simulink model "Fuzzy"  (R2021a)
settings: Solver=VariableStepAuto  StartTime=0.0  StopTime=30  RelTol=1e-3
values from neighbouring files (symbols this model uses):
  K = Kp/(a*Ke)    (= 32)    [code.m]    (also in tester.m)
  Kd = a*Ke    (= 0.0566666666667)    [code.m]    (also in tester.m = 0.0416666666667)
  Ke = 1.5    [code.m]    (also in tester.m)
libraries: simulink x3, fuzblock x1
settings Model: PauseTimes=10  Creator=Administrator  LastModifiedBy=Administrator

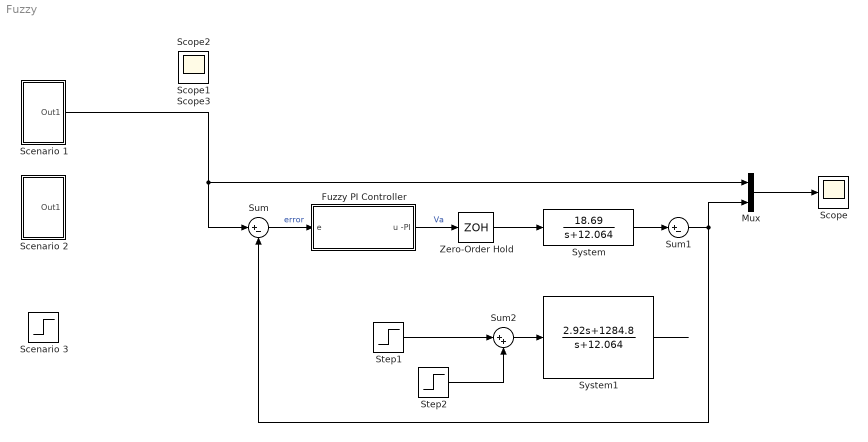
== system Fuzzy ==
  Fuzzy PI Controller : Subsystem
  Mux : Mux  Inputs=2
  "Scenario 1 " : Subsystem
  Scenario 2 : Subsystem
  "Scenario 3 " : Step  Time=0  Before=150  After=150  SampleTime=0
  Scope{,1..3} (4 alike) : Scope
  Step1 : Step  Time=10  Before=0.5  SampleTime=0
  Step2 : Step  Time=20  After=-0.5  SampleTime=0
  Sum : Sum  Inputs=|+-  SampleTime=0.01
  Sum1 : Sum  Inputs=|+-
  Sum2 : Sum  Inputs=|++  SampleTime=0.01
  System : TransferFcn  Numerator=[18.69]  Denominator=[1 12.064]
  System1 : TransferFcn  Numerator=[2.92 1284.8 ]  Denominator=[1 12.064]
  Zero-Order Hold : ZeroOrderHold  SampleTime=0.01
  wires:
  Sum2/1 -> System1/1
  Step1/1 -> Sum2/1
  System/1 -> Sum1/1
  Fuzzy PI Controller/1(u -PI) -> Zero-Order Hold/1  "Va"
  Sum1/1 -> Sum/2, Mux/2
  Sum/1 -> Fuzzy PI Controller/1(e)  "error"
  Mux/1 -> Scope/1
  "Scenario 1 "/1(Out1) -> Sum/1, Mux/1
  Zero-Order Hold/1 -> System/1
  Step2/1 -> Sum2/2
  System1/1 -> ?

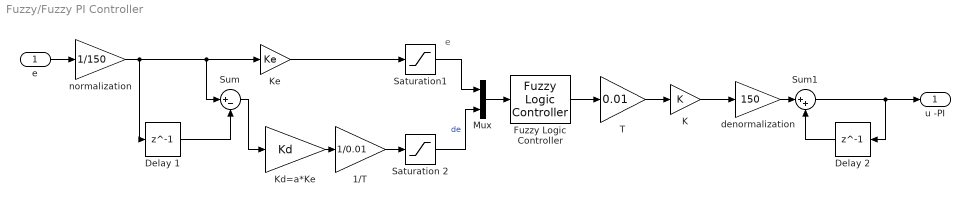
== system Fuzzy/Fuzzy PI Controller ==
  note: e
  e : Inport
  1/T : Gain  Gain=1/0.01  SampleTime=0.01
  Delay 1 : Delay  DelayLength=1  InitialCondition=0  SampleTime=0.01
  Delay 2 : Delay  DelayLength=1  InitialCondition=0  SampleTime=0.01
  Fuzzy Logic Controller : fuzblock/Fuzzy Logic  Controller  FIS='MOTOR.fis'  OutputSampleNumber=101  DataType=double  FuzzifiedInputs=off  RuleFiringStrengths=off  RuleOutputs=off  AggregatedOutputs=off  SimulateUsing=Interpreted execution  OutOfRangeInputValueMessage=warning  NoRuleFiredMessage=warning  EmptyOutputFuzzySetMessage=warning
  K : Gain  Gain=K  SampleTime=0.01
  Kd=a*Ke : Gain  Gain=Kd  SampleTime=0.01
  Ke : Gain  Gain=Ke  SampleTime=0.01
  Mux : Mux  Inputs=2
  Saturation 2 : Saturate  UpperLimit=1  LowerLimit=-1  SampleTime=0.01
  Saturation1 : Saturate  UpperLimit=1  LowerLimit=-1  SampleTime=0.01
  Sum : Sum  Inputs=|+-  SampleTime=0.01
  Sum1 : Sum  Inputs=|++  SampleTime=0.01
  T : Gain  Gain=0.01  SampleTime=0.01
  denormalization : Gain  Gain=150  SampleTime=0.01
  normalization : Gain  Gain=1/150  SampleTime=0.01
  u -PI : Outport
  wires:
  normalization/1 -> Ke/1, Sum/1, Delay 1/1
  Sum/1 -> Kd=a*Ke/1
  Kd=a*Ke/1 -> 1/T/1
  Ke/1 -> Saturation1/1
  1/T/1 -> Saturation 2/1
  Saturation1/1 -> Mux/1
  Saturation 2/1 -> Mux/2  "de"
  Fuzzy Logic Controller/1 -> T/1
  T/1 -> K/1
  K/1 -> denormalization/1
  denormalization/1 -> Sum1/1
  Delay 2/1 -> Sum1/2
  Sum1/1 -> u -PI/1, Delay 2/1
  Mux/1 -> Fuzzy Logic Controller/1
  e/1 -> normalization/1
  Delay 1/1 -> Sum/2

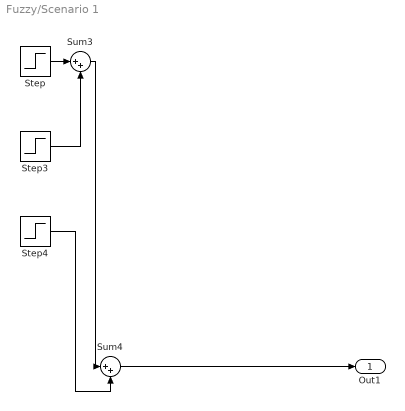
== system Fuzzy/Scenario 1  ==
  Step : Step  Time=0  Before=150  After=150  SampleTime=0
  Step3 : Step  Time=10  After=-50  SampleTime=0
  Step4 : Step  Time=20  After=50  SampleTime=0
  Sum3 : Sum  Inputs=|++
  Sum4 : Sum  Inputs=|++
  Out1 : Outport
  wires:
  Step/1 -> Sum3/1
  Step3/1 -> Sum3/2
  Step4/1 -> Sum4/2
  Sum3/1 -> Sum4/1
  Sum4/1 -> Out1/1

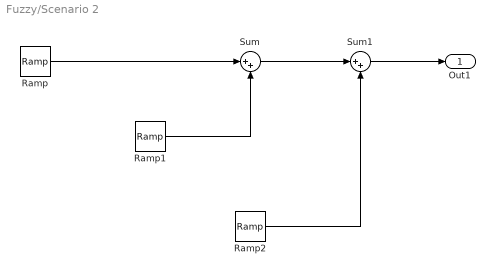
== system Fuzzy/Scenario 2 ==
  Ramp : simulink/Sources/Ramp  slope=15  start=0  InitialOutput=0  VectorParams1D=off
  Ramp1 : simulink/Sources/Ramp  slope=-15  start=10  InitialOutput=0  VectorParams1D=off
  Ramp2 : simulink/Sources/Ramp  slope=-15  start=20  InitialOutput=0  VectorParams1D=off
  Sum : Sum  Inputs=|++
  Sum1 : Sum  Inputs=|++
  Out1 : Outport
  wires:
  Ramp2/1 -> Sum1/2
  Ramp1/1 -> Sum/2
  Sum1/1 -> Out1/1
  Sum/1 -> Sum1/1
  Ramp/1 -> Sum/1
